simulink model "luenberger_observer_case4"  (R2019b)
settings: Solver=VariableStepAuto  StartTime=0.0  StopTime=50  RelTol=1e-3
undefined symbols (not defined in the file): Aob4, Bob4, C4, Cob4, Dob4
settings Model: Creator=Anubhav Paras  LastModifiedBy=Anubhav Paras

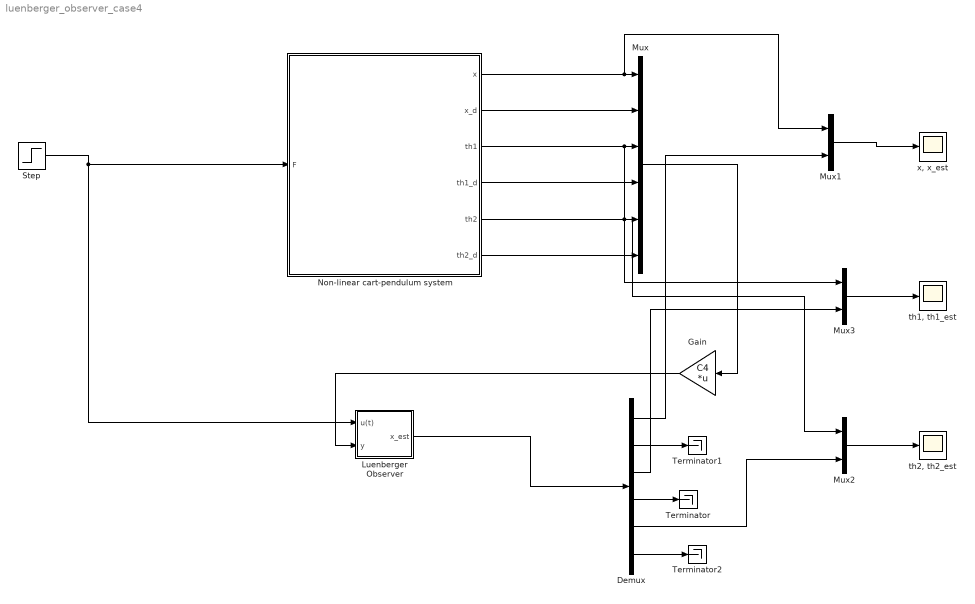
== system luenberger_observer_case4 ==
  " Luenberger Observer" : Subsystem
  " Non-linear cart-pendulum system" : Subsystem
  Demux : Demux  Outputs=6
  Gain : Gain  Gain=C4  Multiplication=Matrix(K*u)
  Mux : Mux  Inputs=6
  Mux1 : Mux  Inputs=2
  Mux2 : Mux  Inputs=2
  Mux3 : Mux  Inputs=2
  Step : Step  SampleTime=0
  Terminator : Terminator
  Terminator1 : Terminator
  Terminator2 : Terminator
  "th1, th1_est" : Scope
  "th2, th2_est" : Scope
  "x, x_est" : Scope
  wires:
  Demux/2 -> Terminator1/1
  Demux/4 -> Terminator/1
  " Luenberger Observer"/1(x_est) -> Demux/1
  Mux2/1 -> "th2, th2_est"/1
  Demux/1 -> Mux1/2
  Mux1/1 -> "x, x_est"/1
  Demux/5 -> Mux2/2
  " Non-linear cart-pendulum system"/2(x_d) -> Mux/2
  " Non-linear cart-pendulum system"/5(th2) -> Mux2/1, Mux/5
  Demux/6 -> Terminator2/1
  " Non-linear cart-pendulum system"/3(th1) -> Mux3/1, Mux/3
  " Non-linear cart-pendulum system"/6(th2_d) -> Mux/6
  Mux3/1 -> "th1, th1_est"/1
  " Non-linear cart-pendulum system"/1(x) -> Mux1/1, Mux/1
  Gain/1 -> " Luenberger Observer"/2(y)
  " Non-linear cart-pendulum system"/4(th1_d) -> Mux/4
  Mux/1 -> Gain/1
  Demux/3 -> Mux3/2
  Step/1 -> " Non-linear cart-pendulum system"/1(F), " Luenberger Observer"/1(u(t))

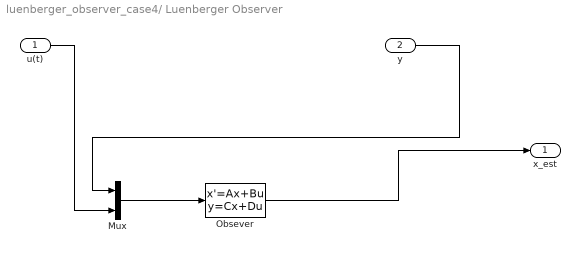
== system luenberger_observer_case4/ Luenberger Observer ==
  u(t) : Inport
  y : Inport  Port=2
  Mux : Mux  Inputs=2
  "Obsever " : StateSpace  A=Aob4  B=Bob4  C=Cob4  D=Dob4  InitialCondition=0
  x_est : Outport
  wires:
  Mux/1 -> "Obsever "/1
  "Obsever "/1 -> x_est/1
  y/1 -> Mux/1
  u(t)/1 -> Mux/2

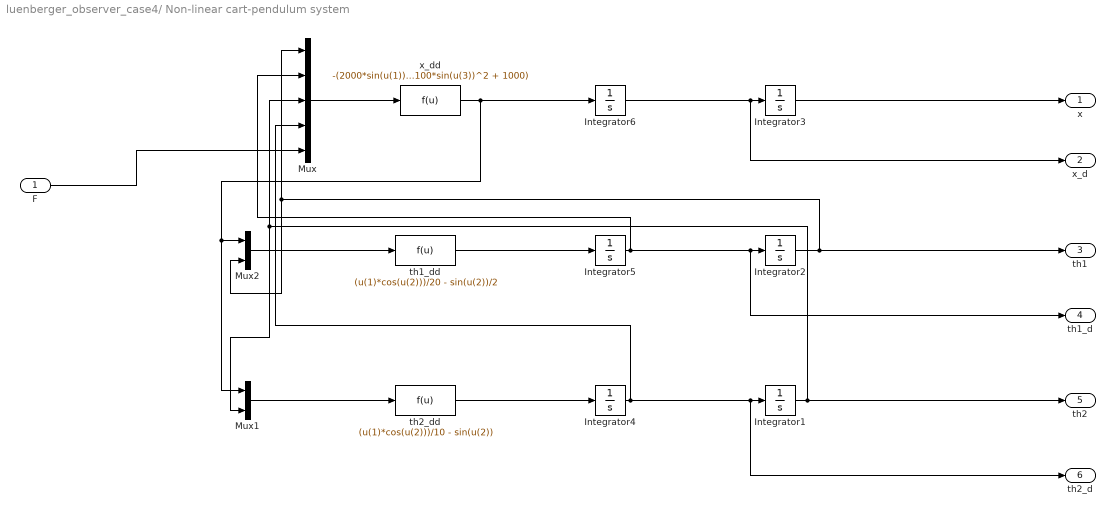
== system luenberger_observer_case4/ Non-linear cart-pendulum system ==
  F : Inport
  Integrator1 : Integrator  InitialCondition=0.1
  Integrator2 : Integrator  InitialCondition=0.1
  Integrator3 : Integrator  InitialCondition=0.5
  Integrator4 : Integrator
  Integrator5 : Integrator
  Integrator6 : Integrator
  Mux : Mux  Inputs=5
  Mux1 : Mux  Inputs=2
  Mux2 : Mux  Inputs=2
  th1_dd : Fcn  Expr=(u(1)*cos(u(2)))/20 - sin(u(2))/2
  th2_dd : Fcn  Expr=(u(1)*cos(u(2)))/10 - sin(u(2))
  x_dd : Fcn  Expr=-(2000*sin(u(1))*u(2)^2 + 1000*sin(u(3))*u(4)^2 - u(5) + 1000*cos(u(1))*sin(u(1)) - 1000*cos(u(3))*sin(u(3)))/(100*sin(u(1))^2 + 100*sin(u(3))^2 + 1000)
  x : Outport
  x_d : Outport  Port=2
  th1 : Outport  Port=3
  th1_d : Outport  Port=4
  th2 : Outport  Port=5
  th2_d : Outport  Port=6
  wires:
  th2_dd/1 -> Integrator4/1
  x_dd/1 -> Mux1/1, Mux2/1, Integrator6/1
  Integrator6/1 -> x_d/1, Integrator3/1
  Mux1/1 -> th2_dd/1
  Integrator5/1 -> Mux/2, th1_d/1, Integrator2/1
  Mux/1 -> x_dd/1
  Integrator1/1 -> th2/1, Mux1/2, Mux/3
  Integrator2/1 -> th1/1, Mux2/2, Mux/1
  th1_dd/1 -> Integrator5/1
  Integrator4/1 -> Mux/4, th2_d/1, Integrator1/1
  Mux2/1 -> th1_dd/1
  Integrator3/1 -> x/1
  F/1 -> Mux/5
